simulink model "practica12022A"  (R2022a)
settings: Solver=FixedStepDiscrete  StartTime=0.0  StopTime=0.2  FixedStep=0.001  RelTol=1e-3
settings Model: Creator=edgar  LastModifiedBy=Anahi Monserrat
settings ModelReferenceCC: EnableRefExpFcnMdlSchedulingChecks=off
settings RTWCC: Description=Generic Real-Time Target

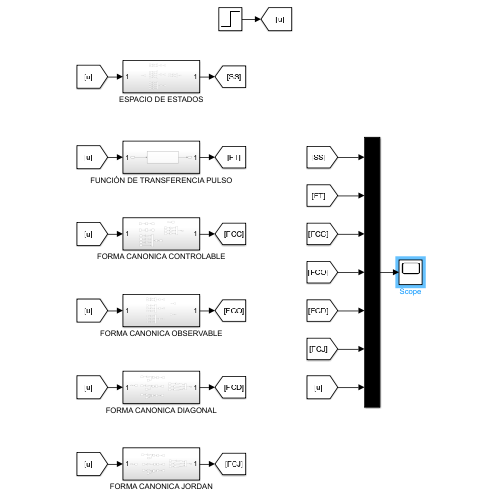
[thumbnail: Simulink's stored preview of the top-level diagram]
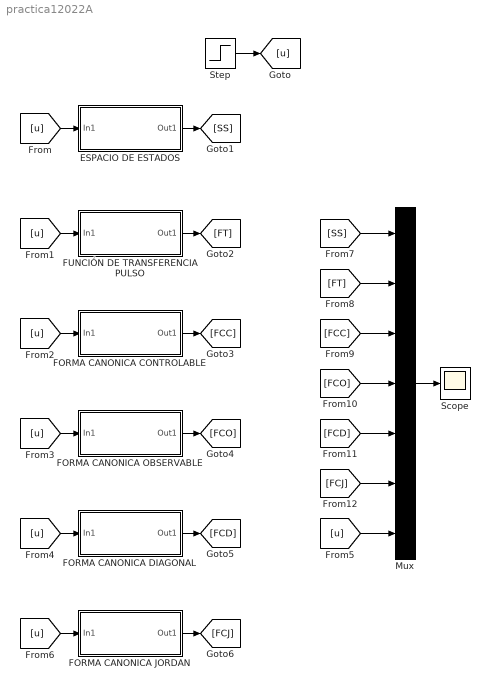
== system practica12022A ==
  ESPACIO DE ESTADOS : Subsystem
  FORMA CANONICA CONTROLABLE : Subsystem
  FORMA CANONICA DIAGONAL : Subsystem
  FORMA CANONICA JORDAN : Subsystem
  FORMA CANONICA OBSERVABLE : Subsystem
  FUNCIÓN DE TRANSFERENCIA PULSO : Subsystem
  Mux : Mux  Inputs=7
  Scope : Scope
  Step : Step  Time=0  SampleTime=0
  wires:
  Step/1 -> [u]
  [u] -> ESPACIO DE ESTADOS/1(In1)
  [u] -> FUNCIÓN DE TRANSFERENCIA PULSO/1(In1)
  [u] -> FORMA CANONICA OBSERVABLE/1(In1)
  [u] -> FORMA CANONICA DIAGONAL/1(In1)
  Mux/1 -> Scope/1
  [u] -> FORMA CANONICA CONTROLABLE/1(In1)
  [u] -> FORMA CANONICA JORDAN/1(In1)
  [SS] -> Mux/1
  ESPACIO DE ESTADOS/1(Out1) -> [SS]
  [FT] -> Mux/2
  [u] -> Mux/7
  FUNCIÓN DE TRANSFERENCIA PULSO/1(Out1) -> [FT]
  FORMA CANONICA CONTROLABLE/1(Out1) -> [FCC]
  FORMA CANONICA OBSERVABLE/1(Out1) -> [FCO]
  FORMA CANONICA DIAGONAL/1(Out1) -> [FCD]
  FORMA CANONICA JORDAN/1(Out1) -> [FCJ]
  [FCC] -> Mux/3
  [FCO] -> Mux/4
  [FCD] -> Mux/5
  [FCJ] -> Mux/6

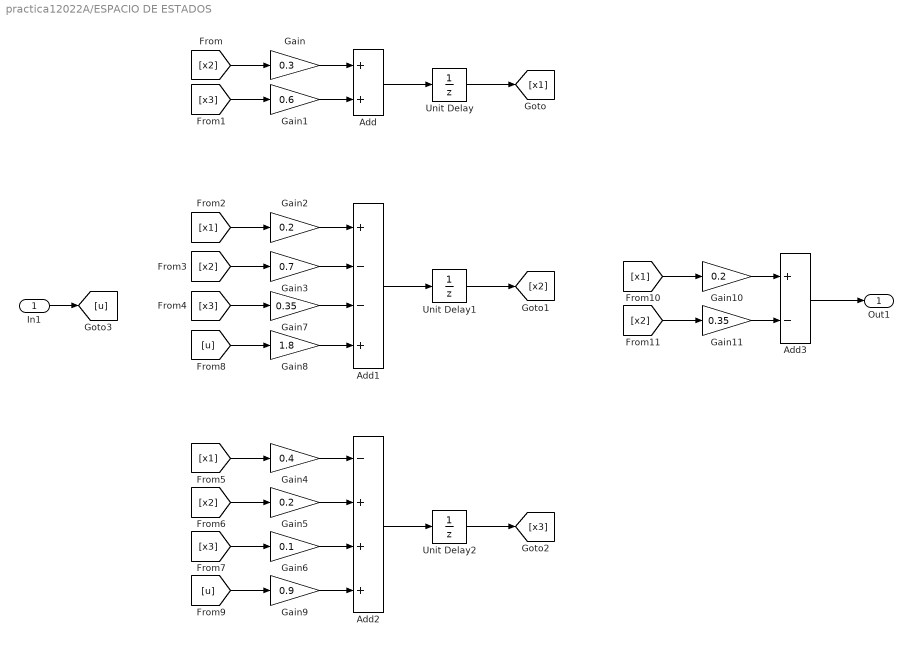
== system practica12022A/ESPACIO DE ESTADOS ==
  In1 : Inport
  Add : Sum
  Add1 : Sum  Inputs=+--+
  Add2 : Sum  Inputs=-+++
  Add3 : Sum  Inputs=+-
  Gain : Gain  Gain=0.3
  Gain1 : Gain  Gain=0.6
  Gain10 : Gain  Gain=0.2
  Gain11 : Gain  Gain=0.35
  Gain2 : Gain  Gain=0.2
  Gain3 : Gain  Gain=0.7
  Gain4 : Gain  Gain=0.4
  Gain5 : Gain  Gain=0.2
  Gain6 : Gain  Gain=0.1
  Gain7 : Gain  Gain=0.35
  Gain8 : Gain  Gain=1.8
  Gain9 : Gain  Gain=0.9
  Unit Delay : UnitDelay  SampleTime=-1  HasFrameUpgradeWarning=on
  Unit Delay1 : UnitDelay  SampleTime=-1  HasFrameUpgradeWarning=on
  Unit Delay2 : UnitDelay  SampleTime=-1  HasFrameUpgradeWarning=on
  Out1 : Outport
  wires:
  Unit Delay/1 -> [x1]
  Unit Delay1/1 -> [x2]
  Unit Delay2/1 -> [x3]
  Add2/1 -> Unit Delay2/1
  Add1/1 -> Unit Delay1/1
  Add/1 -> Unit Delay/1
  Gain/1 -> Add/1
  Gain1/1 -> Add/2
  Gain7/1 -> Add1/3
  Gain3/1 -> Add1/2
  Gain2/1 -> Add1/1
  Gain5/1 -> Add2/2
  Gain4/1 -> Add2/1
  Gain6/1 -> Add2/3
  [x2] -> Gain/1
  [x3] -> Gain1/1
  [x1] -> Gain2/1
  [x2] -> Gain3/1
  [x3] -> Gain7/1
  [x1] -> Gain4/1
  [x2] -> Gain5/1
  [x3] -> Gain6/1
  In1/1 -> [u]
  Gain9/1 -> Add2/4
  [u] -> Gain9/1
  [u] -> Gain8/1
  Gain8/1 -> Add1/4
  Add3/1 -> Out1/1
  [x2] -> Gain11/1
  [x1] -> Gain10/1
  Gain11/1 -> Add3/2
  Gain10/1 -> Add3/1

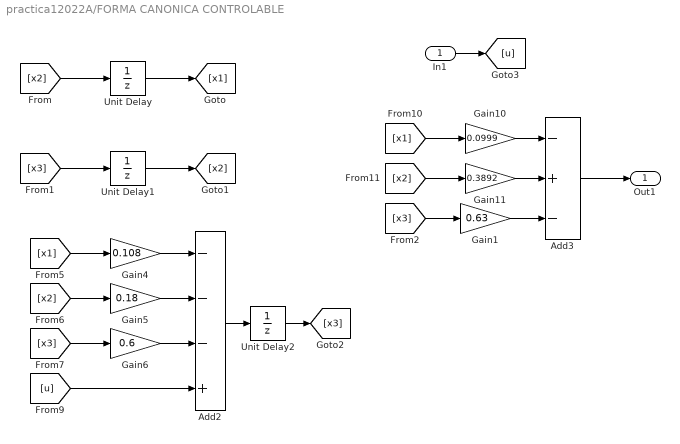
== system practica12022A/FORMA CANONICA CONTROLABLE ==
  In1 : Inport
  Add2 : Sum  Inputs=---+
  Add3 : Sum  Inputs=-+-
  Gain1 : Gain  Gain=0.63
  Gain10 : Gain  Gain=0.0999
  Gain11 : Gain  Gain=0.3892
  Gain4 : Gain  Gain=0.108
  Gain5 : Gain  Gain=0.18
  Gain6 : Gain  Gain=0.6
  Unit Delay : UnitDelay  SampleTime=-1  HasFrameUpgradeWarning=on
  Unit Delay1 : UnitDelay  SampleTime=-1  HasFrameUpgradeWarning=on
  Unit Delay2 : UnitDelay  SampleTime=-1  HasFrameUpgradeWarning=on
  Out1 : Outport
  wires:
  Gain10/1 -> Add3/1
  Gain11/1 -> Add3/2
  [x1] -> Gain10/1
  [x2] -> Gain11/1
  Add3/1 -> Out1/1
  [u] -> Add2/4
  In1/1 -> [u]
  [x3] -> Gain6/1
  [x2] -> Gain5/1
  [x1] -> Gain4/1
  Gain6/1 -> Add2/3
  Gain4/1 -> Add2/1
  Gain5/1 -> Add2/2
  Add2/1 -> Unit Delay2/1
  Unit Delay2/1 -> [x3]
  Unit Delay1/1 -> [x2]
  Unit Delay/1 -> [x1]
  [x2] -> Unit Delay/1
  [x3] -> Unit Delay1/1
  [x3] -> Gain1/1
  Gain1/1 -> Add3/3

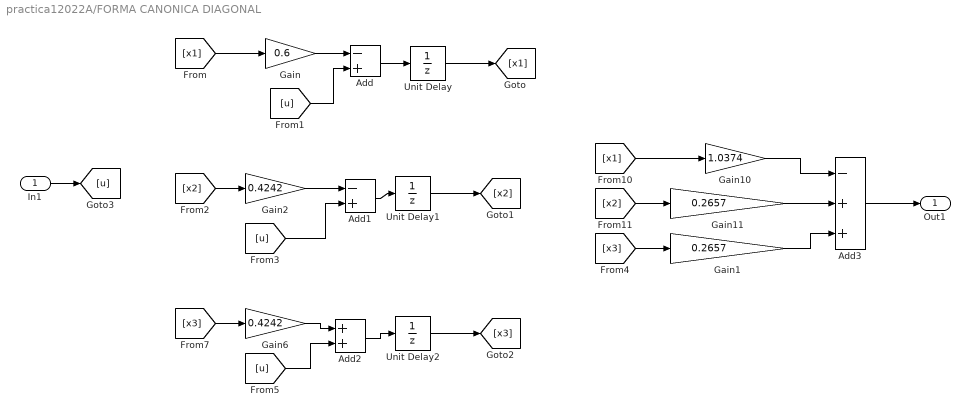
== system practica12022A/FORMA CANONICA DIAGONAL ==
  In1 : Inport
  Add : Sum  Inputs=-+
  Add1 : Sum  Inputs=-+
  Add2 : Sum
  Add3 : Sum  Inputs=-++
  Gain : Gain  Gain=0.6
  Gain1 : Gain  Gain=0.2657  OutDataTypeStr=double
  Gain10 : Gain  Gain=1.0374
  Gain11 : Gain  Gain=0.2657  OutDataTypeStr=double
  Gain2 : Gain  Gain=0.4242
  Gain6 : Gain  Gain=0.4242
  Unit Delay : UnitDelay  SampleTime=-1  HasFrameUpgradeWarning=on
  Unit Delay1 : UnitDelay  SampleTime=-1  HasFrameUpgradeWarning=on
  Unit Delay2 : UnitDelay  SampleTime=-1  HasFrameUpgradeWarning=on
  Out1 : Outport
  wires:
  Gain10/1 -> Add3/1
  Gain11/1 -> Add3/2
  [x1] -> Gain10/1
  [x2] -> Gain11/1
  Add3/1 -> Out1/1
  In1/1 -> [u]
  [x3] -> Gain6/1
  [x2] -> Gain2/1
  Unit Delay2/1 -> [x3]
  Unit Delay1/1 -> [x2]
  Unit Delay/1 -> [x1]
  [x1] -> Gain/1
  Gain/1 -> Add/1
  [u] -> Add/2
  Add/1 -> Unit Delay/1
  Gain2/1 -> Add1/1
  Add2/1 -> Unit Delay2/1
  Gain6/1 -> Add2/1
  Add1/1 -> Unit Delay1/1
  Gain1/1 -> Add3/3
  [x3] -> Gain1/1
  [u] -> Add2/2
  [u] -> Add1/2

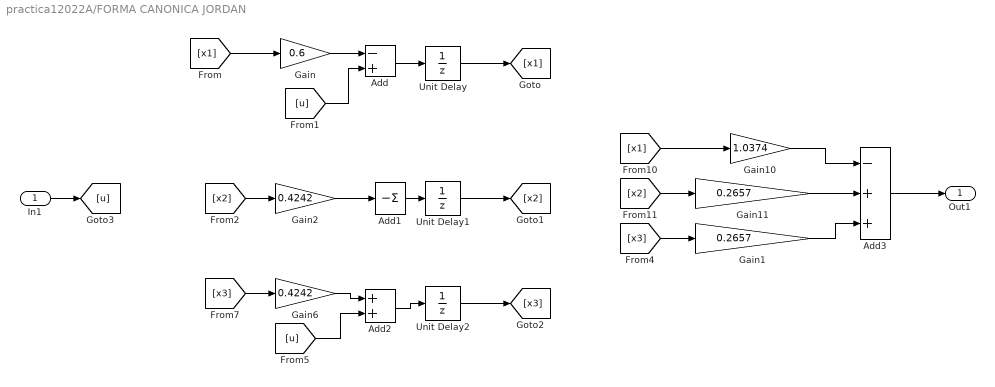
== system practica12022A/FORMA CANONICA JORDAN ==
  In1 : Inport
  Add : Sum  Inputs=-+
  Add1 : Sum  Inputs=-
  Add2 : Sum
  Add3 : Sum  Inputs=-++
  Gain : Gain  Gain=0.6
  Gain1 : Gain  Gain=0.2657  OutDataTypeStr=double
  Gain10 : Gain  Gain=1.0374
  Gain11 : Gain  Gain=0.2657  OutDataTypeStr=double
  Gain2 : Gain  Gain=0.4242
  Gain6 : Gain  Gain=0.4242
  Unit Delay : UnitDelay  SampleTime=-1  HasFrameUpgradeWarning=on
  Unit Delay1 : UnitDelay  SampleTime=-1  HasFrameUpgradeWarning=on
  Unit Delay2 : UnitDelay  SampleTime=-1  HasFrameUpgradeWarning=on
  Out1 : Outport
  wires:
  Gain10/1 -> Add3/1
  Gain11/1 -> Add3/2
  [x1] -> Gain10/1
  [x2] -> Gain11/1
  Add3/1 -> Out1/1
  In1/1 -> [u]
  [x3] -> Gain6/1
  [x2] -> Gain2/1
  Unit Delay2/1 -> [x3]
  Unit Delay1/1 -> [x2]
  Unit Delay/1 -> [x1]
  [x1] -> Gain/1
  Gain/1 -> Add/1
  [u] -> Add/2
  Add/1 -> Unit Delay/1
  Gain2/1 -> Add1/1
  Add2/1 -> Unit Delay2/1
  Gain6/1 -> Add2/1
  Add1/1 -> Unit Delay1/1
  Gain1/1 -> Add3/3
  [x3] -> Gain1/1
  [u] -> Add2/2

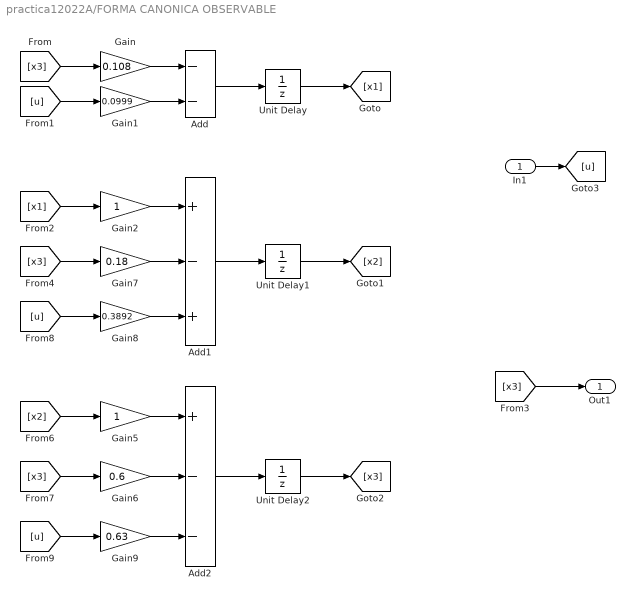
== system practica12022A/FORMA CANONICA OBSERVABLE ==
  In1 : Inport
  Add : Sum  Inputs=--
  Add1 : Sum  Inputs=+-+
  Add2 : Sum  Inputs=+--
  Gain : Gain  Gain=0.108
  Gain1 : Gain  Gain=0.0999
  Gain2 : Gain
  Gain5 : Gain
  Gain6 : Gain  Gain=0.6
  Gain7 : Gain  Gain=0.18
  Gain8 : Gain  Gain=0.3892
  Gain9 : Gain  Gain=0.63
  Unit Delay : UnitDelay  SampleTime=-1  HasFrameUpgradeWarning=on
  Unit Delay1 : UnitDelay  SampleTime=-1  HasFrameUpgradeWarning=on
  Unit Delay2 : UnitDelay  SampleTime=-1  HasFrameUpgradeWarning=on
  Out1 : Outport
  wires:
  Unit Delay/1 -> [x1]
  Unit Delay1/1 -> [x2]
  Unit Delay2/1 -> [x3]
  Add2/1 -> Unit Delay2/1
  Add1/1 -> Unit Delay1/1
  Add/1 -> Unit Delay/1
  Gain/1 -> Add/1
  Gain1/1 -> Add/2
  Gain2/1 -> Add1/1
  [x3] -> Gain/1
  [u] -> Gain1/1
  [x1] -> Gain2/1
  [x3] -> Gain7/1
  [x2] -> Gain5/1
  [x3] -> Gain6/1
  In1/1 -> [u]
  Gain9/1 -> Add2/3
  [u] -> Gain9/1
  [u] -> Gain8/1
  Gain8/1 -> Add1/3
  Gain7/1 -> Add1/2
  Gain5/1 -> Add2/1
  Gain6/1 -> Add2/2
  [x3] -> Out1/1

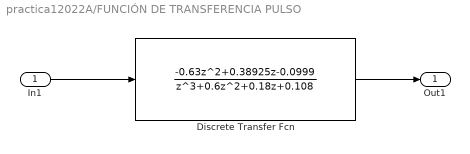
== system practica12022A/FUNCIÓN DE TRANSFERENCIA PULSO ==
  In1 : Inport
  Discrete Transfer Fcn : DiscreteTransferFcn  Numerator=[-0.63 0.38925 -0.0999]  Denominator=[1 0.6 0.18 0.108]
  Out1 : Outport
  wires:
  Discrete Transfer Fcn/1 -> Out1/1
  In1/1 -> Discrete Transfer Fcn/1
